simulink model "ex2"  (R2023b)
settings: Solver=VariableStepAuto  StartTime=0.0  StopTime=10.0  RelTol=1e-3
values from neighbouring files (symbols this model uses):
  T = 0.01    [ex2.m]    (also in ex5.m = 10; listing.m = 0.001)
settings Model: Creator=sorin  LastModifiedBy=sorin

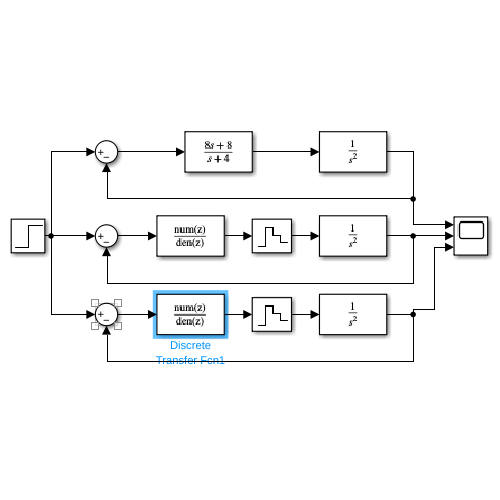
[thumbnail: Simulink's stored preview of the top-level diagram]
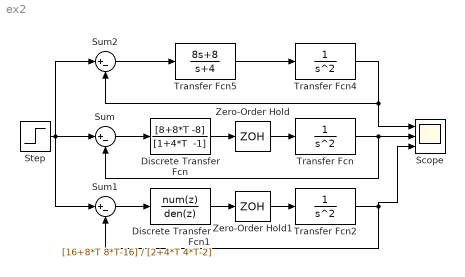
== system ex2 ==
  Discrete Transfer Fcn : DiscreteTransferFcn  Numerator=[8+8*T -8]  Denominator="[1+4*T  -1]"
  Discrete Transfer Fcn1 : DiscreteTransferFcn  Numerator=[16+8*T 8*T-16]  Denominator=[2+4*T 4*T-2]
  Scope : Scope  NumInputPorts=3
  Step : Step  SampleTime=0
  Sum : Sum  Inputs=|+-
  Sum1 : Sum  Inputs=|+-
  Sum2 : Sum  Inputs=|+-
  Transfer Fcn : TransferFcn  Denominator="[1  0 0]"
  Transfer Fcn2 : TransferFcn  Denominator="[1  0 0]"
  Transfer Fcn4 : TransferFcn  Denominator="[1  0 0]"
  Transfer Fcn5 : TransferFcn  Numerator=[8 8]  Denominator=[1 4]
  Zero-Order Hold : ZeroOrderHold  SampleTime=T
  Zero-Order Hold1 : ZeroOrderHold  SampleTime=T
  wires:
  Transfer Fcn/1 -> Sum/2, Scope/2
  Transfer Fcn2/1 -> Scope/3, Sum1/2
  Step/1 -> Sum2/1, Sum/1, Sum1/1
  Transfer Fcn5/1 -> Transfer Fcn4/1
  Sum2/1 -> Transfer Fcn5/1
  Transfer Fcn4/1 -> Scope/1, Sum2/2
  Sum/1 -> Discrete Transfer Fcn/1
  Discrete Transfer Fcn1/1 -> Zero-Order Hold1/1
  Zero-Order Hold1/1 -> Transfer Fcn2/1
  Discrete Transfer Fcn/1 -> Zero-Order Hold/1
  Zero-Order Hold/1 -> Transfer Fcn/1
  Sum1/1 -> Discrete Transfer Fcn1/1
